simulink subsystem "AirframePowertrain"  (R2024b)
settings: Solver=VariableStepAuto  StartTime=0.0  StopTime=10.0  RelTol=1e-3
undefined symbols (not defined in the file): contact, motorPID, percWeightGain, uavParam, windVel
libraries: mbdriLib x3, aerolibasang x2, fl_lib x1, nesl_utility x1
settings Model: Creator=jjha  LastModifiedBy=jjha
settings RTWCC: GPUComputeCapability=3.5

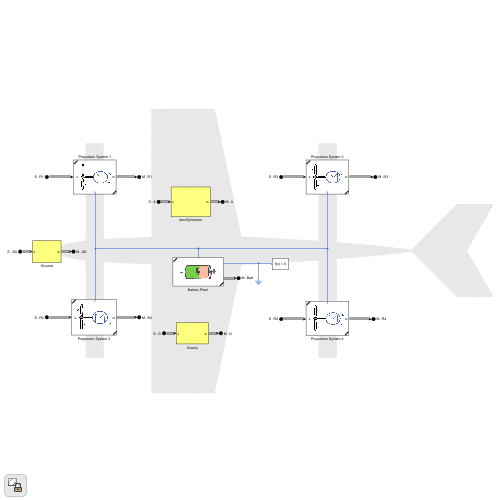
[thumbnail: Simulink's stored preview of the top-level diagram]
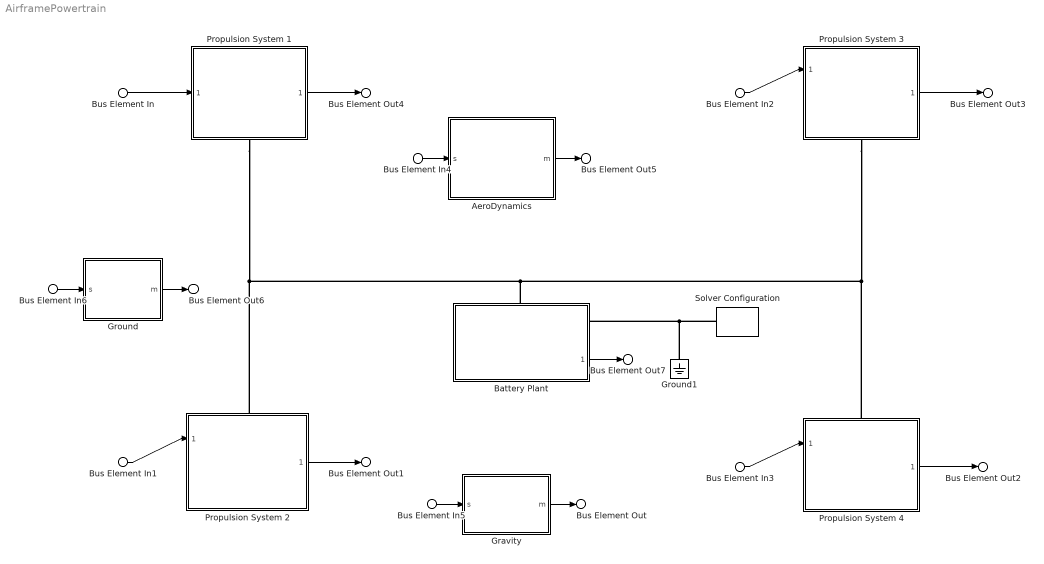
== system AirframePowertrain ==
  Bus Element In : Inport  PortName=S  Element=R1
  Bus Element In1 : Inport  PortName=S  Element=R2
  Bus Element In2 : Inport  PortName=S  Element=R3
  Bus Element In3 : Inport  PortName=S  Element=R4
  Bus Element In4 : Inport  PortName=S  Element=A
  Bus Element In5 : Inport  PortName=S  Element=G
  Bus Element In6 : Inport  PortName=S  Element=AD
  AeroDynamics : Subsystem
  Battery Plant : Subsystem  ReferencedSubsystem=BatteryPlantModel_Table
      settings: PortSchema="{\"entries\":[{\"content\":{\"sides\":[{\"content\":{\"connectorIds\":[\"LConn1\"]},\"type\":\"ConnectorPlacement.EquallySpacedRectSide\",\"uuid\":\"ba36f307-b33b-4535-ba0b-2e0bfd99fc4d\"},{\"content\":{\"connectorIds\":[\"RConn2\",\"Out1\"],\"side\":\"RIGHT\"},\"type\":\"ConnectorPlacement.EquallySpacedRectSide\",\"uuid\":\"89704593-04c2-4c1a-a3b9-13b3f56a74b5\"},{\"content\":{\"connectorIds\":[\"RConn1\"],\"side\":\"TOP\"},\"type\":\"ConnectorPlacement.EquallySpacedRectSide\",\"uuid\":\"1daeac74-7d2b-4aa4-8837-06dc1649b516\"},{\"content\":{\"side\":\"BOTTOM\"},\"type\":\"ConnectorPlacement.EquallySpacedRectSide\",\"uuid\":\"a55355a8-f534-49c8-a897-d3f7ff506222\"}]},\"type\":\"ConnectorPlacement.EquallySpacedConnector\",\"uuid\":\"2c693ef8-3b08-48d7-935c-b55223a280fc\"}],\"packageUris\":[\"http://schema.mathworks.com/mf0/Connector/R2020b\"],\"version\":\"1.0\"}"
  Gravity : Subsystem
  Ground : Subsystem
  Ground1 : fl_lib/Electrical/Electrical Elements/Electrical Reference
  Propulsion System 1 : Subsystem  ReferencedSubsystem=PropulsionSystem  RotorArm=uavParam.geom.RotorArm1  Kp=motorPID.Kpp  Ki=motorPID.Kii  Kd=motorPID.Kdd  N=motorPID.N
      settings: PortSchema="{\"entries\":[{\"content\":{\"sides\":[{\"content\":{\"connectorIds\":[\"In1\"]},\"type\":\"ConnectorPlacement.EquallySpacedRectSide\",\"uuid\":\"a75aafe4-98d2-4ab0-9654-1a116df6472c\"},{\"content\":{\"connectorIds\":[\"Out1\"],\"side\":\"RIGHT\"},\"type\":\"ConnectorPlacement.EquallySpacedRectSide\",\"uuid\":\"2075eb3f-d81d-4e0c-b871-39ed3a8467db\"},{\"content\":{\"side\":\"TOP\"},\"type\":\"ConnectorPlacement.EquallySpacedRectSide\",\"uuid\":\"9db392e5-d372-4f9a-b849-10c0fd16bebf\"},{\"content\":{\"connectorIds\":[\"RConn1\"],\"side\":\"BOTTOM\"},\"type\":\"ConnectorPlacement.EquallySpacedRectSide\",\"uuid\":\"0cb625c0-fbe4-4004-9810-4dcf6ffdfbe8\"}]},\"type\":\"ConnectorPlacement.EquallySpacedConnector\",\"uuid\":\"a89763ad-9d11-48f7-8f0c-3b7b7595f410\"}],\"packageUris\":[\"http://schema.mathworks.com/mf0/Connector/R2020b\"],\"version\":\"1.0\"}"
  Propulsion System 2 : Subsystem  ReferencedSubsystem=PropulsionSystem  RotorArm=uavParam.geom.RotorArm2  Kp=motorPID.Kpp  Ki=motorPID.Kii  Kd=motorPID.Kdd  N=motorPID.N
      settings: PortSchema="{\"entries\":[{\"content\":{\"sides\":[{\"content\":{\"connectorIds\":[\"In1\",\"LConn1\"]},\"type\":\"ConnectorPlacement.EquallySpacedRectSide\",\"uuid\":\"a75aafe4-98d2-4ab0-9654-1a116df6472c\"},{\"content\":{\"connectorIds\":[\"Out1\"],\"side\":\"RIGHT\"},\"type\":\"ConnectorPlacement.EquallySpacedRectSide\",\"uuid\":\"2075eb3f-d81d-4e0c-b871-39ed3a8467db\"},{\"content\":{\"connectorIds\":[\"RConn1\"],\"side\":\"TOP\"},\"type\":\"ConnectorPlacement.EquallySpacedRectSide\",\"uuid\":\"9db392e5-d372-4f9a-b849-10c0fd16bebf\"}]},\"type\":\"ConnectorPlacement.EquallySpacedConnector\",\"uuid\":\"a89763ad-9d11-48f7-8f0c-3b7b7595f410\"}],\"packageUris\":[\"http://schema.mathworks.com/mf0/Connector/R2020b\"],\"version\":\"1.0\"}"
  Propulsion System 3 : Subsystem  ReferencedSubsystem=PropulsionSystem  RotorArm=uavParam.geom.RotorArm3  Kp=motorPID.Kpp  Ki=motorPID.Kii  Kd=motorPID.Kdd  N=motorPID.N
      settings: PortSchema="{\"entries\":[{\"content\":{\"sides\":[{\"content\":{\"connectorIds\":[\"In1\",\"LConn1\"]},\"type\":\"ConnectorPlacement.EquallySpacedRectSide\",\"uuid\":\"a75aafe4-98d2-4ab0-9654-1a116df6472c\"},{\"content\":{\"connectorIds\":[\"Out1\"],\"side\":\"RIGHT\"},\"type\":\"ConnectorPlacement.EquallySpacedRectSide\",\"uuid\":\"2075eb3f-d81d-4e0c-b871-39ed3a8467db\"},{\"content\":{\"side\":\"TOP\"},\"type\":\"ConnectorPlacement.EquallySpacedRectSide\",\"uuid\":\"9db392e5-d372-4f9a-b849-10c0fd16bebf\"},{\"content\":{\"connectorIds\":[\"RConn1\"],\"side\":\"BOTTOM\"},\"type\":\"ConnectorPlacement.EquallySpacedRectSide\",\"uuid\":\"14e310fc-3705-44ea-ab02-95783124972c\"}]},\"type\":\"ConnectorPlacement.EquallySpacedConnector\",\"uuid\":\"a89763ad-9d11-48f7-8f0c-3b7b7595f410\"}],\"packageUris\":[\"http://schema.mathworks.com/mf0/Connector/R2020b\"],\"version\":\"1.0\"}"
  Propulsion System 4 : Subsystem  ReferencedSubsystem=PropulsionSystem  RotorArm=uavParam.geom.RotorArm4  Kp=motorPID.Kpp  Ki=motorPID.Kii  Kd=motorPID.Kdd  N=motorPID.N
      settings: PortSchema="{\"entries\":[{\"content\":{\"sides\":[{\"content\":{\"connectorIds\":[\"In1\",\"LConn1\"]},\"type\":\"ConnectorPlacement.EquallySpacedRectSide\",\"uuid\":\"a75aafe4-98d2-4ab0-9654-1a116df6472c\"},{\"content\":{\"connectorIds\":[\"Out1\"],\"side\":\"RIGHT\"},\"type\":\"ConnectorPlacement.EquallySpacedRectSide\",\"uuid\":\"2075eb3f-d81d-4e0c-b871-39ed3a8467db\"},{\"content\":{\"connectorIds\":[\"RConn1\"],\"side\":\"TOP\"},\"type\":\"ConnectorPlacement.EquallySpacedRectSide\",\"uuid\":\"9db392e5-d372-4f9a-b849-10c0fd16bebf\"}]},\"type\":\"ConnectorPlacement.EquallySpacedConnector\",\"uuid\":\"a89763ad-9d11-48f7-8f0c-3b7b7595f410\"}],\"packageUris\":[\"http://schema.mathworks.com/mf0/Connector/R2020b\"],\"version\":\"1.0\"}"
  Solver Configuration : nesl_utility/Solver Configuration  PhysicalDomain=network_engine_domain  SubClassName=solver  LeftPortType=input  RightPortType=generic  Tones=[]  Harmonics=[]  SimulateNoise=off  Profile=off  UseLocalSampling=off  EnableSwitchedLinearOptims=on  FrequencyDomain=off  UseCCode=off  RelTol=0.001  AbsTol=0.001  MinStep=1e-09  ToWorkspace=off  RevertToSquareIcSolve=off  NumHomotopyIterations=100  PhasorMode=off  PhasorModeNumHarmonics=1  ConsistencySolver=NEWTON_XTOL_AFTER_FTOL  IndexReductionMethod=DerivativeReplacement  DoDC=off  ResidualTolerance=1e-09  ConsistencyTolSource=GLOBAL  ConsistencyAbsTol=0.001  ConsistencyRelTol=0.001  ConsistencyTolFactor=0.001  UseLocalSolver=on  LocalSolverChoice=NE_BACKWARD_EULER_ADVANCER  ResolveIndetEquations=on  FunctionEvalNumThread=1  LocalSolverSampleTime=0.01  DoFixedCost=off  MaxNonlinIter=3  MaxModeIter=2  ComputeImpulses=off  ImpulseIterations=2  LinearAlgebra=auto  LinearAlgebraNumThread=0  EquationFormulation=NE_TIME_EF  DelaysMemoryBudget=1024  AutomaticFiltering=on  FilteringTimeConstant=0.001  PartitionStorageMethod=AS_NEEDED  PartitionMemoryBudget=1024  PartitionMethod=ROBUST  MultibodyUseLocalSolver=off  MultibodyLocalSolverChoice=ODE1  MultibodyLocalSolverSampleTime=0.001
  Bus Element Out : Outport  PortName=M  Element=G
  Bus Element Out1 : Outport  PortName=M  Element=R2
  Bus Element Out2 : Outport  PortName=M  Element=R4
  Bus Element Out3 : Outport  PortName=M  Element=R3
  Bus Element Out4 : Outport  PortName=M  Element=R1
  Bus Element Out5 : Outport  PortName=M  Element=A
  Bus Element Out6 : Outport  PortName=M  Element=AD
  Bus Element Out7 : Outport  PortName=M  Element=Batt
  wires:
  Bus Element In1/1 -> Propulsion System 2/1
  Bus Element In2/1 -> Propulsion System 3/1
  Bus Element In3/1 -> Propulsion System 4/1
  Bus Element In/1 -> Propulsion System 1/1
  Bus Element In4/1 -> AeroDynamics/1(s)
  Bus Element In5/1 -> Gravity/1(s)
  Gravity/1(m) -> Bus Element Out/1
  Propulsion System 2/1 -> Bus Element Out1/1
  Propulsion System 4/1 -> Bus Element Out2/1
  Propulsion System 3/1 -> Bus Element Out3/1
  Propulsion System 1/1 -> Bus Element Out4/1
  AeroDynamics/1(m) -> Bus Element Out5/1
  Bus Element In6/1 -> Ground/1(s)
  Ground/1(m) -> Bus Element Out6/1
  Battery Plant/1 -> Bus Element Out7/1
  connections:
  Propulsion System 3/RConn1 -- Propulsion System 1/RConn1 -- Propulsion System 2/RConn1 -- Battery Plant/RConn1 -- Propulsion System 4/RConn1
  Solver Configuration/RConn1 -- Ground1/LConn1 -- Battery Plant/RConn2

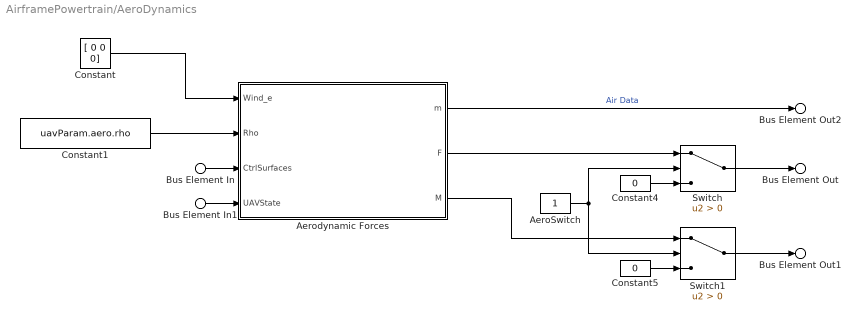
== system AirframePowertrain/AeroDynamics ==
  Bus Element In : Inport  PortName=s  Element=Ctrl
  Bus Element In1 : Inport  PortName=s  Element=St
  AeroSwitch : Constant
  Aerodynamic Forces : Subsystem
  Constant : Constant  Value=[ 0 0 0]
      settings: AttributesFormatString=%<Value>
  Constant1 : Constant  Value=uavParam.aero.rho
  Constant4 : Constant  Value=0
  Constant5 : Constant  Value=0
  Switch : Switch  Criteria=u2 > Threshold  SaturateOnIntegerOverflow=off  InputSameDT=off
  Switch1 : Switch  Criteria=u2 > Threshold  SaturateOnIntegerOverflow=off  InputSameDT=off
  Bus Element Out : Outport  PortName=m  Element=Force
  Bus Element Out1 : Outport  PortName=m  Element=Moment
  Bus Element Out2 : Outport  PortName=m  Element=AirData
  wires:
  Bus Element In1/1 -> Aerodynamic Forces/4(UAVState)
  Bus Element In/1 -> Aerodynamic Forces/3(CtrlSurfaces)
  Constant4/1 -> Switch/3
  Aerodynamic Forces/3(M) -> Switch1/1
  Aerodynamic Forces/2(F) -> Switch/1
  Constant5/1 -> Switch1/3
  AeroSwitch/1 -> Switch/2, Switch1/2
  Constant/1 -> Aerodynamic Forces/1(Wind_e)
  Constant1/1 -> Aerodynamic Forces/2(Rho)
  Aerodynamic Forces/1(m) -> Bus Element Out2/1  "Air Data"
  Switch/1 -> Bus Element Out/1
  Switch1/1 -> Bus Element Out1/1

== system AirframePowertrain/Gravity ==
  Bus Element In : Inport  PortName=s  Element=DCMbe
  Constant : Constant  Value=[0 0 uavParam.aero.g]'
  Gain : Gain  Gain=uavParam.geom.mass*percWeightGain
  Matrix Multiply : Product  Multiplication=Matrix(*)
  Bus Element Out : Outport  PortName=m  Element=gravityForce
  wires:
  Bus Element In/1 -> Matrix Multiply/1
  Constant/1 -> Matrix Multiply/2
  Matrix Multiply/1 -> Gain/1
  Gain/1 -> Bus Element Out/1  "Gravity Force"

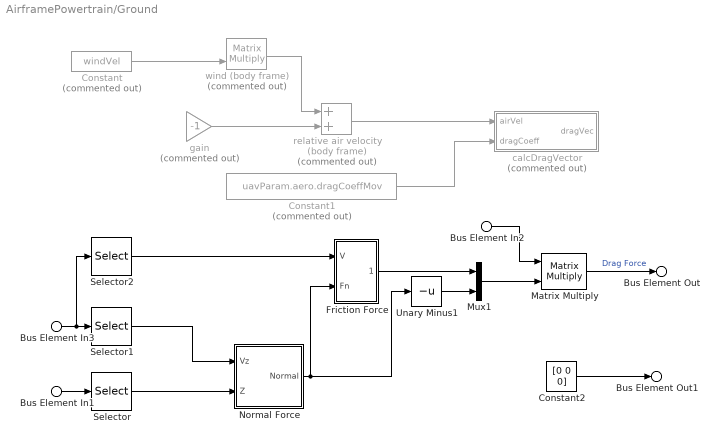
== system AirframePowertrain/Ground ==
  Bus Element In2 : Inport  PortName=s  Element=DCMbe
  Bus Element In3 : Inport  PortName=s  Element=Ve
  Bus Element In1 : Inport  PortName=s  Element=Xe
  Constant : Constant  Commented=on  Value=windVel
  Constant1 : Constant  Commented=on  Value=uavParam.aero.dragCoeffMov
  Constant2 : Constant  Value=[0 0 0]  SampleTime=-1
  Friction Force : Subsystem
  Matrix Multiply : Product  Multiplication=Matrix(*)
  Mux1 : Mux  Inputs=2
  Normal Force : Subsystem
  Selector : Selector  InputPortWidth=3  IndexOptions=Index vector (dialog)  Indices=[3]  OutputSizes=1
  Selector1 : Selector  InputPortWidth=3  IndexOptions=Index vector (dialog)  Indices=[3]  OutputSizes=1
  Selector2 : Selector  InputPortWidth=3  IndexOptions=Index vector (dialog)  Indices=[1,2]  OutputSizes=1
  Unary Minus1 : UnaryMinus
  calcDragVector : MATLAB Function  Commented=on  TreatAsAtomicUnit=on
  gain : Gain  Commented=on  Gain=-1
  relative air velocity (body frame) : Sum  Commented=on
  wind (body frame) : Product  Commented=on  Multiplication=Matrix(*)
  Bus Element Out : Outport  PortName=m  Element=GroundForce
  Bus Element Out1 : Outport  PortName=m  Element=GroundMoment
  wires:
  Normal Force/1(Normal) -> Unary Minus1/1, Friction Force/2(Fn)
  Selector1/1 -> Normal Force/1(Vz)
  Constant2/1 -> Bus Element Out1/1
  Selector/1 -> Normal Force/2(Z)
  Unary Minus1/1 -> Mux1/2
  Bus Element In1/1 -> Selector/1
  Mux1/1 -> Matrix Multiply/2
  Friction Force/1(Friction) -> Mux1/1
  Bus Element In2/1 -> Matrix Multiply/1
  Bus Element In3/1 -> Selector1/1, Selector2/1
  Selector2/1 -> Friction Force/1(V)
  ? -> gain/1
  relative air velocity (body frame)/1 -> calcDragVector/1(airVel)
  gain/1 -> relative air velocity (body frame)/2
  Constant1/1 -> calcDragVector/2(dragCoeff)
  Constant/1 -> wind (body frame)/2
  wind (body frame)/1 -> relative air velocity (body frame)/1
  Matrix Multiply/1 -> Bus Element Out/1  "Drag Force"

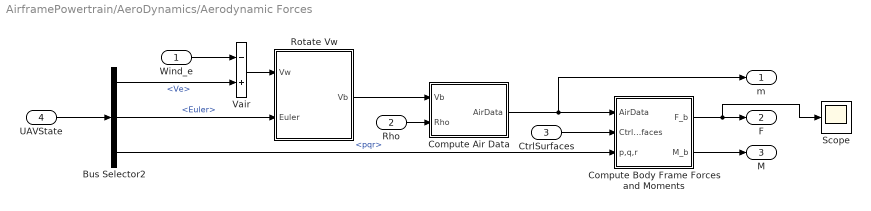
== system AirframePowertrain/AeroDynamics/Aerodynamic Forces ==
  Wind_e : Inport
  Rho : Inport  Port=2
  CtrlSurfaces : Inport  Port=3
  UAVState : Inport  Port=4
  Bus Selector2 : BusSelector  OutputSignals=Ve,Euler,pqr
  Compute Air Data : Subsystem  TreatAsAtomicUnit=on  VariantControl=use_aerospace_blocks == 1
  Compute Body Frame Forces and Moments : Subsystem
  Rotate Vw : Subsystem
  Scope : Scope
  Vair : Sum  Inputs=-+  InputSameDT=on  SaturateOnIntegerOverflow=on  OutDataTypeStr=Inherit: Same as first input
  m : Outport  VectorParamsAs1DForOutWhenUnconnected=off
  F : Outport  Port=2
  M : Outport  Port=3
  wires:
  Vair/1 -> Rotate Vw/1(Vw)
  Bus Selector2/2 -> Rotate Vw/2(Euler)  "<Euler>"
  Rho/1 -> Compute Air Data/2(Rho)
  Rotate Vw/1(Vb) -> Compute Air Data/1(Vb)
  Compute Body Frame Forces and Moments/2(M_b) -> M/1
  Bus Selector2/3 -> Compute Body Frame Forces and Moments/3(p,q,r)  "<pqr>"
  Compute Air Data/1(AirData) -> Compute Body Frame Forces and Moments/1(AirData), m/1
  CtrlSurfaces/1 -> Compute Body Frame Forces and Moments/2(CtrlSurfaces)
  Wind_e/1 -> Vair/1
  Compute Body Frame Forces and Moments/1(F_b) -> F/1, Scope/1
  UAVState/1 -> Bus Selector2/1
  Bus Selector2/1 -> Vair/2  "<Ve>"

== system AirframePowertrain/Ground/Friction Force ==
  V : Inport
  Fn : Inport  Port=2
  Product : Product
  Soft Coulomb Friction : Subsystem
  Unary Minus : UnaryMinus
  Friction : Outport
  wires:
  V/1 -> Soft Coulomb Friction/1(V)
  Product/1 -> Unary Minus/1
  Soft Coulomb Friction/1(Out1) -> Product/1
  Fn/1 -> Product/2
  Unary Minus/1 -> Friction/1

== system AirframePowertrain/Ground/Normal Force ==
  Vz : Inport
  Z : Inport  Port=2
  Add : Sum
  Constant : Constant  Value=0  SampleTime=-1
  Damper : Gain  Gain=-sqrt(contact.spring*uavParam.geom.mass)
  Saturation : Saturate  UpperLimit=inf  LowerLimit=0  ZeroCross=off
  Spring Kp : Gain  Gain=-contact.spring
  Switch : Switch  Criteria=u2 > Threshold  SaturateOnIntegerOverflow=off  InputSameDT=off
  Unary Minus : UnaryMinus
  Unary Minus1 : UnaryMinus
  Normal : Outport
  wires:
  Unary Minus1/1 -> Damper/1
  Unary Minus/1 -> Switch/2, Spring Kp/1
  Saturation/1 -> Normal/1
  Vz/1 -> Unary Minus1/1
  Spring Kp/1 -> Add/1
  Damper/1 -> Add/2
  Switch/1 -> Saturation/1
  Z/1 -> Unary Minus/1
  Constant/1 -> Switch/1
  Add/1 -> Switch/3

== system AirframePowertrain/AeroDynamics/Aerodynamic Forces/Compute Air Data ==
  Vb : Inport  PortDimensions=3
  Rho : Inport  Port=2
  Add : Sum
  Bus Creator : BusCreator  Inputs=4
  Constant : Constant  Value=5/57.296
  Dynamic Pressure : aerolibasang/Dynamic Pressure
  Gain : Gain
  "Incidence, Sideslip, & Airspeed" : aerolibasang/Incidence, Sideslip, & Airspeed
  Saturation : Saturate  UpperLimit=14*pi/180  LowerLimit=-14*pi/180
  To Workspace : ToWorkspace  VariableName=Alpha  SaveFormat=Timeseries  SampleTime=-1
  AirData : Outport  VectorParamsAs1DForOutWhenUnconnected=off
  wires:
  Add/1 -> Gain/1  "alpha"
  Gain/1 -> To Workspace/1
  Constant/1 -> Add/1
  "Incidence, Sideslip, & Airspeed"/1 -> Bus Creator/1, Add/2  "alpha"
  Saturation/1 -> Bus Creator/2  "beta"
  "Incidence, Sideslip, & Airspeed"/2 -> Saturation/1  "beta"
  Vb/1 -> Dynamic Pressure/1, "Incidence, Sideslip, & Airspeed"/1
  Dynamic Pressure/1 -> Bus Creator/4  "q"
  "Incidence, Sideslip, & Airspeed"/3 -> Bus Creator/3  "airspeed"
  Rho/1 -> Dynamic Pressure/2
  Bus Creator/1 -> AirData/1

== system AirframePowertrain/AeroDynamics/Aerodynamic Forces/Compute Body Frame Forces and Moments ==
  AirData : Inport
  CtrlSurfaces : Inport  Port=2
  p,q,r : Inport  Port=3
  Bus Selector : BusSelector  OutputSignals=alpha,beta
  Mux : Mux  Inputs=2
  Rotate FM to body frame : Subsystem
  Wind frame F& M : Subsystem
  F_b : Outport  Unit=kg*m/s^2  VectorParamsAs1DForOutWhenUnconnected=off
  M_b : Outport  Port=2  Unit=kg*m/s  VectorParamsAs1DForOutWhenUnconnected=off
  wires:
  AirData/1 -> Bus Selector/1, Wind frame F& M/1(Airdata)
  CtrlSurfaces/1 -> Wind frame F& M/2(CtrlSurfaces)
  Rotate FM to body frame/1(F_b) -> F_b/1
  Rotate FM to body frame/2(M_b) -> M_b/1
  p,q,r/1 -> Wind frame F& M/3(p,q,r)
  Wind frame F& M/1(FM_w) -> Rotate FM to body frame/1(FM_w)  "FM_W"
  Bus Selector/1 -> Mux/1  "<alpha>"
  Bus Selector/2 -> Mux/2  "<beta>"
  Mux/1 -> Rotate FM to body frame/2(alpha_beta)

== system AirframePowertrain/AeroDynamics/Aerodynamic Forces/Rotate Vw ==
  Vw : Inport
  Euler : Inport  Port=2
  RL2B : mbdriLib/Coordinates/RL2B  SystemSampleTime=-1  VariantActivationTime=update diagram  AllowFlexibleInterface=on  Latency=0  AutoFrameSizeCalculation=off
  RL2B * Vw : Product  Multiplication=Matrix(*)  InputSameDT=on  SaturateOnIntegerOverflow=on  OutDataTypeStr=Inherit: Same as first input
  Vb : Outport  Unit=m/s  VectorParamsAs1DForOutWhenUnconnected=off
  wires:
  Euler/1 -> RL2B/1
  RL2B/1 -> RL2B * Vw/1
  Vw/1 -> RL2B * Vw/2
  RL2B * Vw/1 -> Vb/1

== system AirframePowertrain/Ground/Friction Force/Soft Coulomb Friction ==
  note: Pennestrì, E., Rossi, V., Salvini, P. et al. Review and comparison of dry friction force models. Nonlinear Dyn 83, 1785–1801 (2016). https://doi.org/10.1007/s11071-015-2485-3
  V : Inport
  Tanh : Trigonometry  Operator=tanh
  friction coefficient : Gain  Gain=contact.rollingFriction*1.2
  vd : Gain  Gain=1/contact.vd
  Out1 : Outport
  wires:
  friction coefficient/1 -> Out1/1
  Tanh/1 -> friction coefficient/1
  vd/1 -> Tanh/1
  V/1 -> vd/1

== system AirframePowertrain/AeroDynamics/Aerodynamic Forces/Compute Body Frame Forces and Moments/Rotate FM to body frame ==
  FM_w : Inport
  alpha_beta : Inport  Port=2
  Forces : Selector  InputPortWidth=6  IndexOptions=Index vector (dialog)  Indices=[1 2 3]  OutputSizes=[(-2)]
  Moments : Selector  InputPortWidth=6  IndexOptions=Index vector (dialog)  Indices=[4 5 6]  OutputSizes=[(-2)]
  Rotate Forces : Subsystem
  Rotate Moments : Subsystem
  F_b : Outport  VectorParamsAs1DForOutWhenUnconnected=off
  M_b : Outport  Port=2  VectorParamsAs1DForOutWhenUnconnected=off
  wires:
  Rotate Forces/1(F_b) -> F_b/1
  Rotate Moments/1(M_b) -> M_b/1
  Forces/1 -> Rotate Forces/1(F_w)
  FM_w/1 -> Forces/1, Moments/1
  Moments/1 -> Rotate Moments/2(M_w)
  alpha_beta/1 -> Rotate Moments/1(alpha_beta), Rotate Forces/2(alpha_beta)

== system AirframePowertrain/AeroDynamics/Aerodynamic Forces/Compute Body Frame Forces and Moments/Wind frame F& M ==
  Airdata : Inport
  CtrlSurfaces : Inport  Port=2
  p,q,r : Inport  Port=3
  Bus Creator1 : BusCreator  Inputs=2
  Bus Selector1 : BusSelector  OutputSignals=dA,dR
  Bus Selector2 : BusSelector  OutputSignals=dE,dA,dR
  Bus Selector6 : BusSelector  OutputSignals=beta,airspeed
  Bus Selector7 : BusSelector  OutputSignals=alpha,airspeed
  Get Forces and Moments : Subsystem
  Lateral Channel : Subsystem
  Longitudinal Channel : Subsystem
  FM_w : Outport  PortDimensions=6  VectorParamsAs1DForOutWhenUnconnected=off
  wires:
  Bus Selector2/3 -> Longitudinal Channel/6(dR)  "<dR>"
  Bus Selector2/2 -> Longitudinal Channel/5(dA)  "<dA>"
  Longitudinal Channel/1(Longitudinal) -> Bus Creator1/2
  Lateral Channel/1(Lateral) -> Bus Creator1/1
  p,q,r/1 -> Longitudinal Channel/4(p,q,r), Lateral Channel/5(p,q,r)
  CtrlSurfaces/1 -> Bus Selector2/1, Bus Selector1/1
  Bus Selector1/1 -> Lateral Channel/3(dA)  "<dA>"
  Bus Selector1/2 -> Lateral Channel/4(dR)  "<dR>"
  Bus Selector2/1 -> Longitudinal Channel/3(dE)  "<dE>"
  Airdata/1 -> Get Forces and Moments/1(Airdata), Bus Selector7/1, Bus Selector6/1
  Bus Selector6/1 -> Lateral Channel/1(beta)  "<beta>"
  Bus Selector6/2 -> Lateral Channel/2(Airspeed)  "<airspeed>"
  Bus Selector7/1 -> Longitudinal Channel/1(alpha)  "<alpha>"
  Bus Selector7/2 -> Longitudinal Channel/2(Airpseed)  "<airspeed>"
  Bus Creator1/1 -> Get Forces and Moments/2(AeroCoeffs)
  Get Forces and Moments/1(FM_w) -> FM_w/1

== system AirframePowertrain/AeroDynamics/Aerodynamic Forces/Compute Body Frame Forces and Moments/Rotate FM to body frame/Rotate Forces ==
  F_w : Inport
  alpha_beta : Inport  Port=2
  Product2 : Product  Multiplication=Matrix(*)  SaturateOnIntegerOverflow=on  OutDataTypeStr=Inherit: Same as first input
  RB2W : Subsystem
  RW2B : Math  Operator=transpose  SignedPower=on
  F_b : Outport  PortDimensions=3  VectorParamsAs1DForOutWhenUnconnected=off
  wires:
  RB2W/1(Rw2b) -> RW2B/1
  alpha_beta/1 -> RB2W/1(aoa beta)
  Product2/1 -> F_b/1
  F_w/1 -> Product2/2
  RW2B/1 -> Product2/1

== system AirframePowertrain/AeroDynamics/Aerodynamic Forces/Compute Body Frame Forces and Moments/Rotate FM to body frame/Rotate Moments ==
  alpha_beta : Inport
  M_w : Inport  Port=2
  Product2 : Product  Multiplication=Matrix(*)  SaturateOnIntegerOverflow=on  OutDataTypeStr=Inherit: Same as first input
  RB2W : Subsystem
  RW2B : Math  Operator=transpose  SignedPower=on
  M_b : Outport  PortDimensions=3  VectorParamsAs1DForOutWhenUnconnected=off
  wires:
  M_w/1 -> Product2/2
  Product2/1 -> M_b/1
  alpha_beta/1 -> RB2W/1(aoa beta)
  RB2W/1(Rw2b) -> RW2B/1
  RW2B/1 -> Product2/1

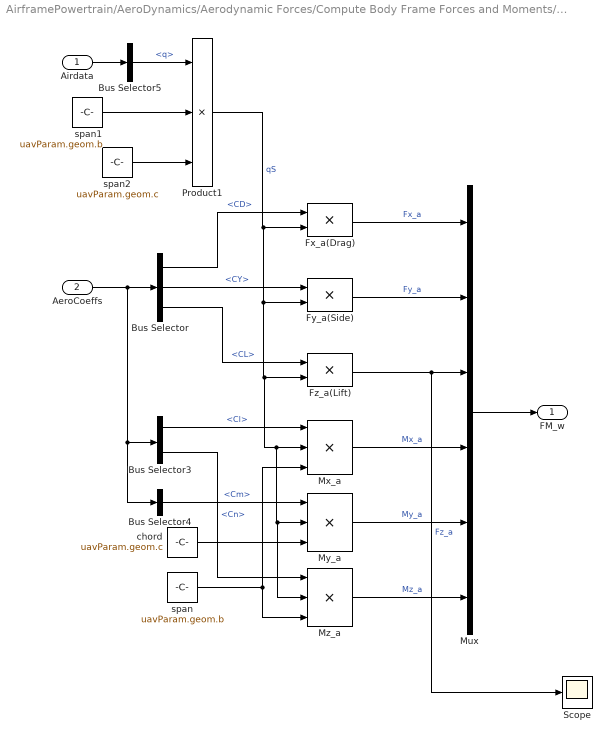
== system AirframePowertrain/AeroDynamics/Aerodynamic Forces/Compute Body Frame Forces and Moments/Wind frame F& M/Get Forces and Moments ==
  Airdata : Inport
  AeroCoeffs : Inport  Port=2
  Bus Selector : BusSelector  OutputSignals=signal2.CD,signal1.CY,signal2.CL
  Bus Selector3 : BusSelector  OutputSignals=signal1.Cl,signal1.Cn
  Bus Selector4 : BusSelector  OutputSignals=signal2.Cm
  Bus Selector5 : BusSelector  OutputSignals=q
  Fx_a(Drag) : Product  Inputs=**  SaturateOnIntegerOverflow=on  OutDataTypeStr=Inherit: Same as first input
  Fy_a(Side) : Product  SaturateOnIntegerOverflow=on  OutDataTypeStr=Inherit: Same as first input
  Fz_a(Lift) : Product  SaturateOnIntegerOverflow=on  OutDataTypeStr=Inherit: Same as first input
  Mux : Mux  Inputs=6
  Mx_a : Product  Inputs=3  SaturateOnIntegerOverflow=on  OutDataTypeStr=Inherit: Same as first input
  My_a : Product  Inputs=3  SaturateOnIntegerOverflow=on  OutDataTypeStr=Inherit: Same as first input
  Mz_a : Product  Inputs=3  SaturateOnIntegerOverflow=on  OutDataTypeStr=Inherit: Same as first input
  Product1 : Product  Inputs=3  SaturateOnIntegerOverflow=on  OutDataTypeStr=Inherit: Same as first input
  Scope : Scope
  chord : Constant  Value=uavParam.geom.c  VectorParams1D=off
      settings: AttributesFormatString=%<Value>
  span : Constant  Value=uavParam.geom.b  VectorParams1D=off
      settings: AttributesFormatString=%<Value>
  span1 : Constant  Value=uavParam.geom.b  VectorParams1D=off
      settings: AttributesFormatString=%<Value>
  span2 : Constant  Value=uavParam.geom.c  VectorParams1D=off
      settings: AttributesFormatString=%<Value>
  FM_w : Outport  VectorParamsAs1DForOutWhenUnconnected=off
  wires:
  Bus Selector5/1 -> Product1/1  "<q>"
  Bus Selector3/1 -> Mx_a/1  "<Cl>"
  span1/1 -> Product1/2
  Product1/1 -> Mz_a/2, My_a/2, Mx_a/2, Fz_a(Lift)/2, Fy_a(Side)/2, Fx_a(Drag)/2  "qS"
  Bus Selector/3 -> Fz_a(Lift)/1  "<CL>"
  Bus Selector3/2 -> Mz_a/1  "<Cn>"
  Mux/1 -> FM_w/1
  Fy_a(Side)/1 -> Mux/2  "Fy_a"
  span/1 -> Mx_a/3, Mz_a/3
  chord/1 -> My_a/3
  Airdata/1 -> Bus Selector5/1
  Mz_a/1 -> Mux/6  "Mz_a"
  Fz_a(Lift)/1 -> Mux/3, Scope/1  "Fz_a"
  My_a/1 -> Mux/5  "My_a"
  AeroCoeffs/1 -> Bus Selector3/1, Bus Selector4/1, Bus Selector/1
  Bus Selector/1 -> Fx_a(Drag)/1  "<CD>"
  Fx_a(Drag)/1 -> Mux/1  "Fx_a"
  span2/1 -> Product1/3
  Bus Selector4/1 -> My_a/1  "<Cm>"
  Bus Selector/2 -> Fy_a(Side)/1  "<CY>"
  Mx_a/1 -> Mux/4  "Mx_a"

== system AirframePowertrain/AeroDynamics/Aerodynamic Forces/Compute Body Frame Forces and Moments/Wind frame F& M/Lateral Channel ==
  beta : Inport
  Airspeed : Inport  Port=2
  dA : Inport  Port=3
  dR : Inport  Port=4
  p,q,r : Inport  Port=5
  Bus Creator : BusCreator  Inputs=3
  CY : Subsystem
  Cl : Subsystem
  Cn : Subsystem
  Lateral : Outport  VectorParamsAs1DForOutWhenUnconnected=off
  wires:
  Bus Creator/1 -> Lateral/1
  CY/1(CY) -> Bus Creator/1  "CY"
  Cn/1(Cn) -> Bus Creator/3  "Cn"
  beta/1 -> Cn/1(beta), Cl/1(beta), CY/1(beta)
  dA/1 -> Cn/2(dA), Cl/2(dA)
  dR/1 -> Cn/3(dR), Cl/3(dR), CY/2(dR)
  Airspeed/1 -> Cl/5(Airspeed), Cn/5(Airspeed), CY/4(Airspeed)
  p,q,r/1 -> CY/3(p,q,r), Cl/4(p,q,r), Cn/4(p,q,r)
  Cl/1(Cl) -> Bus Creator/2  "Cl"

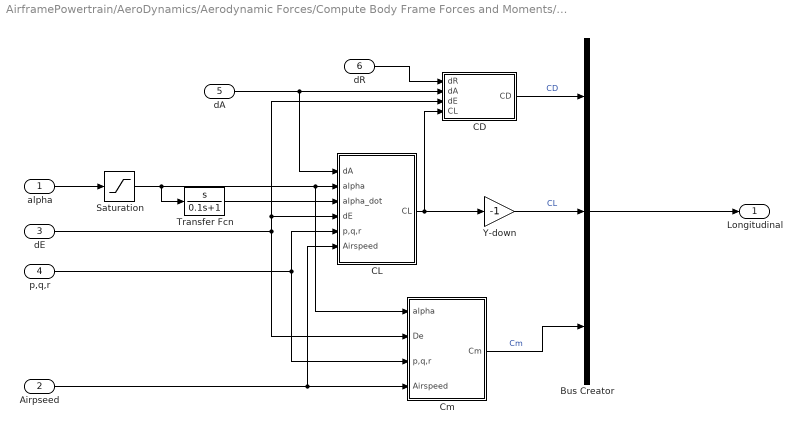
== system AirframePowertrain/AeroDynamics/Aerodynamic Forces/Compute Body Frame Forces and Moments/Wind frame F& M/Longitudinal Channel ==
  alpha : Inport
  Airpseed : Inport  Port=2
  dE : Inport  Port=3
  p,q,r : Inport  Port=4
  dA : Inport  Port=5
  dR : Inport  Port=6
  Bus Creator : BusCreator  Inputs=3
  CD : Subsystem
  CL : Subsystem
  Cm : Subsystem
  Saturation : Saturate  UpperLimit=14*pi/180  LowerLimit=-14*pi/180
  Transfer Fcn : TransferFcn  Numerator=[1 0]  Denominator=[0.1 1]
  Y-down : Gain  Gain=-1  SaturateOnIntegerOverflow=on  OutDataTypeStr=Inherit: Same as input  ParamDataTypeStr=Inherit: Same as input
      settings: AttributesFormatString=%<Gain>
  Longitudinal : Outport  VectorParamsAs1DForOutWhenUnconnected=off
  wires:
  Saturation/1 -> Cm/1(alpha), CL/2(alpha), Transfer Fcn/1
  dA/1 -> CD/2(dA), CL/1(dA)
  dR/1 -> CD/1(dR)
  alpha/1 -> Saturation/1
  CD/1(CD) -> Bus Creator/1  "CD"
  Y-down/1 -> Bus Creator/2  "CL"
  dE/1 -> Cm/2(De), CL/4(dE), CD/3(dE)
  CL/1(CL) -> CD/4(CL), Y-down/1
  Cm/1(Cm) -> Bus Creator/3  "Cm"
  Bus Creator/1 -> Longitudinal/1
  p,q,r/1 -> Cm/3(p,q,r), CL/5(p,q,r)
  Airpseed/1 -> Cm/4(Airspeed), CL/6(Airspeed)
  Transfer Fcn/1 -> CL/3(alpha_dot)

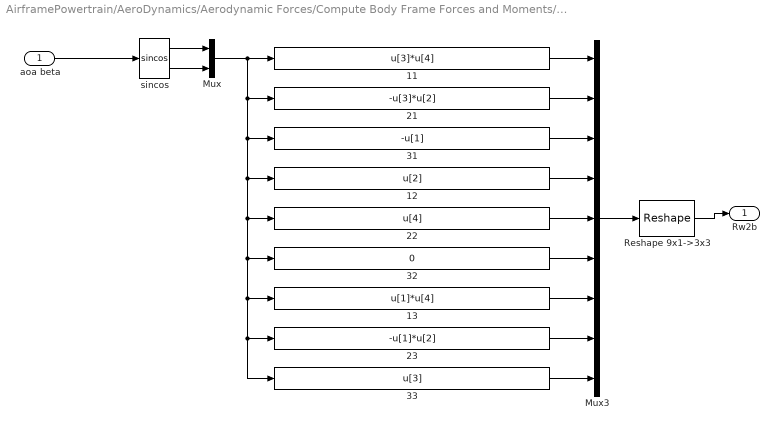
== system AirframePowertrain/AeroDynamics/Aerodynamic Forces/Compute Body Frame Forces and Moments/Rotate FM to body frame/Rotate Forces/RB2W ==
  aoa beta : Inport
  11 : Fcn  Expr=u[3]*u[4]
  12 : Fcn  Expr=u[2]
  13 : Fcn  Expr=u[1]*u[4]
  21 : Fcn  Expr=-u[3]*u[2]
  22 : Fcn  Expr=u[4]
  23 : Fcn  Expr=-u[1]*u[2]
  31 : Fcn  Expr=-u[1]
  32 : Fcn  Expr=0
  33 : Fcn  Expr=u[3]
  Mux : Mux  Inputs=2
  Mux3 : Mux  Inputs=9
  Reshape 9x1->3x3 : Reshape  OutputDimensionality=Customize  OutputDimensions=[3,3]
  sincos : Trigonometry  Operator=sincos
  Rw2b : Outport  VectorParamsAs1DForOutWhenUnconnected=off
  wires:
  Mux3/1 -> Reshape 9x1->3x3/1
  Reshape 9x1->3x3/1 -> Rw2b/1
  11/1 -> Mux3/1
  21/1 -> Mux3/2
  31/1 -> Mux3/3
  12/1 -> Mux3/4
  22/1 -> Mux3/5
  32/1 -> Mux3/6
  13/1 -> Mux3/7
  23/1 -> Mux3/8
  33/1 -> Mux3/9
  sincos/1 -> Mux/1
  sincos/2 -> Mux/2
  aoa beta/1 -> sincos/1
  Mux/1 -> 33/1, 23/1, 13/1, 32/1, 22/1, 12/1, 31/1, 21/1, 11/1

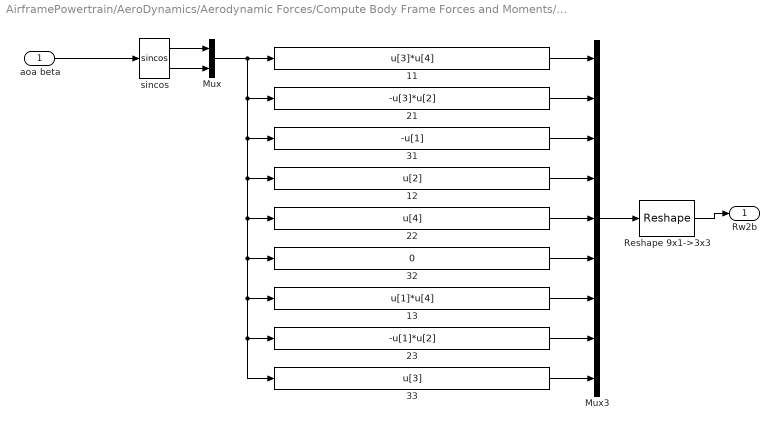
== system AirframePowertrain/AeroDynamics/Aerodynamic Forces/Compute Body Frame Forces and Moments/Rotate FM to body frame/Rotate Moments/RB2W ==
  aoa beta : Inport
  11 : Fcn  Expr=u[3]*u[4]
  12 : Fcn  Expr=u[2]
  13 : Fcn  Expr=u[1]*u[4]
  21 : Fcn  Expr=-u[3]*u[2]
  22 : Fcn  Expr=u[4]
  23 : Fcn  Expr=-u[1]*u[2]
  31 : Fcn  Expr=-u[1]
  32 : Fcn  Expr=0
  33 : Fcn  Expr=u[3]
  Mux : Mux  Inputs=2
  Mux3 : Mux  Inputs=9
  Reshape 9x1->3x3 : Reshape  OutputDimensionality=Customize  OutputDimensions=[3,3]
  sincos : Trigonometry  Operator=sincos
  Rw2b : Outport  VectorParamsAs1DForOutWhenUnconnected=off
  wires:
  Mux3/1 -> Reshape 9x1->3x3/1
  Reshape 9x1->3x3/1 -> Rw2b/1
  11/1 -> Mux3/1
  21/1 -> Mux3/2
  31/1 -> Mux3/3
  12/1 -> Mux3/4
  22/1 -> Mux3/5
  32/1 -> Mux3/6
  13/1 -> Mux3/7
  23/1 -> Mux3/8
  33/1 -> Mux3/9
  sincos/1 -> Mux/1
  sincos/2 -> Mux/2
  aoa beta/1 -> sincos/1
  Mux/1 -> 33/1, 23/1, 13/1, 32/1, 22/1, 12/1, 31/1, 21/1, 11/1

== system AirframePowertrain/AeroDynamics/Aerodynamic Forces/Compute Body Frame Forces and Moments/Wind frame F& M/Lateral Channel/CY ==
  beta : Inport
  dR : Inport  Port=2
  p,q,r : Inport  Port=3
  Airspeed : Inport  Port=4
  CYDr : Constant  Value=uavParam.aero.CYDr
      settings: AttributesFormatString=%<Value>
  CYb : Constant  Value=uavParam.aero.CYb
      settings: AttributesFormatString=%<Value>
  Product : Product  SaturateOnIntegerOverflow=on  OutDataTypeStr=Inherit: Same as first input
  Product1 : Product  SaturateOnIntegerOverflow=on  OutDataTypeStr=Inherit: Same as first input
  Sum2 : Sum  Inputs=++++  SaturateOnIntegerOverflow=on
  roll factors : Subsystem
  CY : Outport  VectorParamsAs1DForOutWhenUnconnected=off
  wires:
  roll factors/2(CYr) -> Sum2/4
  roll factors/1(CYp) -> Sum2/3
  p,q,r/1 -> roll factors/1(p,q,r)
  Airspeed/1 -> roll factors/2(Airspeed)
  Sum2/1 -> CY/1
  CYb/1 -> Product/1
  beta/1 -> Product/2
  Product/1 -> Sum2/1
  CYDr/1 -> Product1/1
  dR/1 -> Product1/2
  Product1/1 -> Sum2/2

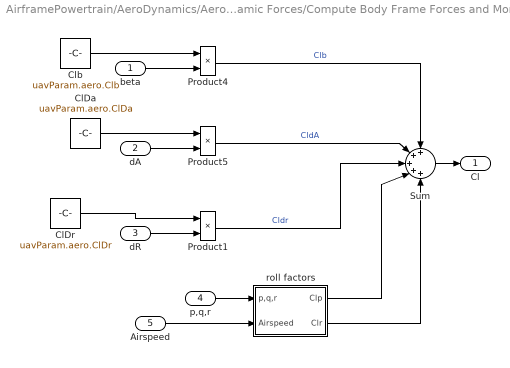
== system AirframePowertrain/AeroDynamics/Aerodynamic Forces/Compute Body Frame Forces and Moments/Wind frame F& M/Lateral Channel/Cl ==
  beta : Inport
  dA : Inport  Port=2
  dR : Inport  Port=3
  p,q,r : Inport  Port=4
  Airspeed : Inport  Port=5
  ClDa : Constant  Value=uavParam.aero.ClDa
      settings: AttributesFormatString=%<Value>
  ClDr : Constant  Value=uavParam.aero.ClDr
      settings: AttributesFormatString=%<Value>
  Clb : Constant  Value=uavParam.aero.Clb
      settings: AttributesFormatString=%<Value>
  Product1 : Product  SaturateOnIntegerOverflow=on  OutDataTypeStr=Inherit: Same as first input
  Product4 : Product  SaturateOnIntegerOverflow=on  OutDataTypeStr=Inherit: Same as first input
  Product5 : Product  SaturateOnIntegerOverflow=on  OutDataTypeStr=Inherit: Same as first input
  Sum : Sum  Inputs=+++++  SaturateOnIntegerOverflow=on
  roll factors : Subsystem
  Cl : Outport  VectorParamsAs1DForOutWhenUnconnected=off
  wires:
  Clb/1 -> Product4/1
  beta/1 -> Product4/2
  ClDa/1 -> Product5/1
  dA/1 -> Product5/2
  ClDr/1 -> Product1/1
  dR/1 -> Product1/2
  Sum/1 -> Cl/1
  Product4/1 -> Sum/1  "Clb"
  Product1/1 -> Sum/3  "Cldr"
  roll factors/2(Clr) -> Sum/5
  p,q,r/1 -> roll factors/1(p,q,r)
  Airspeed/1 -> roll factors/2(Airspeed)
  Product5/1 -> Sum/2  "CldA"
  roll factors/1(Clp) -> Sum/4

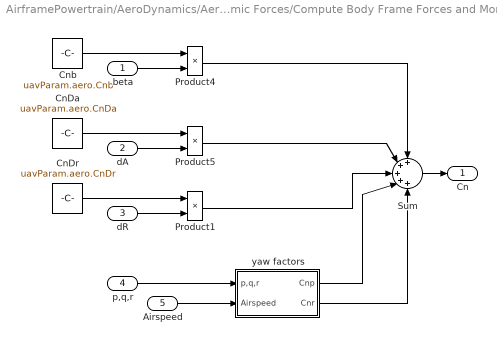
== system AirframePowertrain/AeroDynamics/Aerodynamic Forces/Compute Body Frame Forces and Moments/Wind frame F& M/Lateral Channel/Cn ==
  beta : Inport
  dA : Inport  Port=2
  dR : Inport  Port=3
  p,q,r : Inport  Port=4
  Airspeed : Inport  Port=5
  CnDa : Constant  Value=uavParam.aero.CnDa
      settings: AttributesFormatString=%<Value>
  CnDr : Constant  Value=uavParam.aero.CnDr
      settings: AttributesFormatString=%<Value>
  Cnb : Constant  Value=uavParam.aero.Cnb
      settings: AttributesFormatString=%<Value>
  Product1 : Product  SaturateOnIntegerOverflow=on  OutDataTypeStr=Inherit: Same as first input
  Product4 : Product  SaturateOnIntegerOverflow=on  OutDataTypeStr=Inherit: Same as first input
  Product5 : Product  SaturateOnIntegerOverflow=on  OutDataTypeStr=Inherit: Same as first input
  Sum : Sum  Inputs=+++++  SaturateOnIntegerOverflow=on
  yaw factors : Subsystem
  Cn : Outport  VectorParamsAs1DForOutWhenUnconnected=off
  wires:
  Product4/1 -> Sum/1
  yaw factors/1(Cnp) -> Sum/4
  yaw factors/2(Cnr) -> Sum/5
  Product1/1 -> Sum/3
  Sum/1 -> Cn/1
  dR/1 -> Product1/2
  CnDr/1 -> Product1/1
  dA/1 -> Product5/2
  Product5/1 -> Sum/2
  CnDa/1 -> Product5/1
  beta/1 -> Product4/2
  Cnb/1 -> Product4/1
  p,q,r/1 -> yaw factors/1(p,q,r)
  Airspeed/1 -> yaw factors/2(Airspeed)

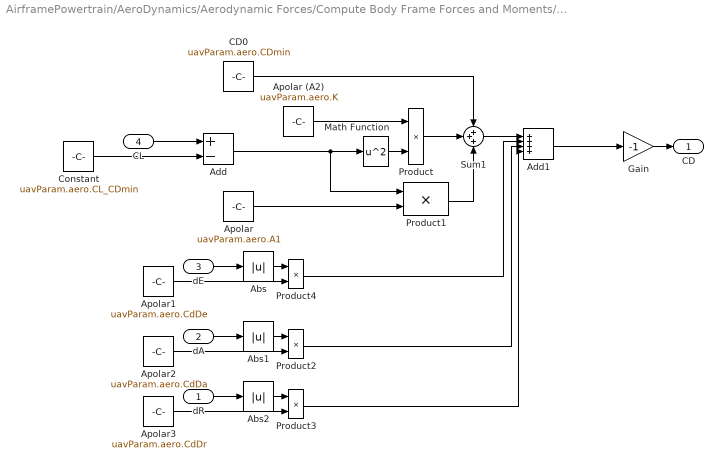
== system AirframePowertrain/AeroDynamics/Aerodynamic Forces/Compute Body Frame Forces and Moments/Wind frame F& M/Longitudinal Channel/CD ==
  dR : Inport
  dA : Inport  Port=2
  dE : Inport  Port=3
  CL : Inport  Port=4
  Abs : Abs  SaturateOnIntegerOverflow=off
  Abs1 : Abs  SaturateOnIntegerOverflow=off
  Abs2 : Abs  SaturateOnIntegerOverflow=off
  Add : Sum  Inputs=+-
  Add1 : Sum  Inputs=++++
  Apolar : Constant  Value=uavParam.aero.A1
      settings: AttributesFormatString=%<Value>
  Apolar (A2) : Constant  Value=uavParam.aero.K
      settings: AttributesFormatString=%<Value>
  Apolar1 : Constant  Value=uavParam.aero.CdDe
      settings: AttributesFormatString=%<Value>
  Apolar2 : Constant  Value=uavParam.aero.CdDa
      settings: AttributesFormatString=%<Value>
  Apolar3 : Constant  Value=uavParam.aero.CdDr
      settings: AttributesFormatString=%<Value>
  CD0 : Constant  Value=uavParam.aero.CDmin
      settings: AttributesFormatString=%<Value>
  Constant : Constant  Value=uavParam.aero.CL_CDmin
  Gain : Gain  Gain=-1  SaturateOnIntegerOverflow=on  OutDataTypeStr=Inherit: Same as input  ParamDataTypeStr=Inherit: Same as input
      settings: AttributesFormatString=%<Gain>
  Math Function : Math  Operator=square  SignedPower=on
  Product{,1..4} (5 alike) : Product  SaturateOnIntegerOverflow=on  OutDataTypeStr=Inherit: Same as first input
  Sum1 : Sum  Inputs=+++  SaturateOnIntegerOverflow=on
  CD : Outport  VectorParamsAs1DForOutWhenUnconnected=off
  wires:
  Product3/1 -> Add1/4
  Product2/1 -> Add1/3
  Product4/1 -> Add1/2
  Add1/1 -> Gain/1
  Sum1/1 -> Add1/1
  dR/1 -> Abs2/1
  Apolar3/1 -> Product3/2
  Abs2/1 -> Product3/1
  dA/1 -> Abs1/1
  Apolar2/1 -> Product2/2
  Abs1/1 -> Product2/1
  Abs/1 -> Product4/1
  dE/1 -> Abs/1
  Apolar1/1 -> Product4/2
  Constant/1 -> Add/2
  CL/1 -> Add/1
  Apolar/1 -> Product1/2
  CD0/1 -> Sum1/1
  Add/1 -> Math Function/1, Product1/1
  Product/1 -> Sum1/2
  Product1/1 -> Sum1/3
  Math Function/1 -> Product/2
  Apolar (A2)/1 -> Product/1
  Gain/1 -> CD/1

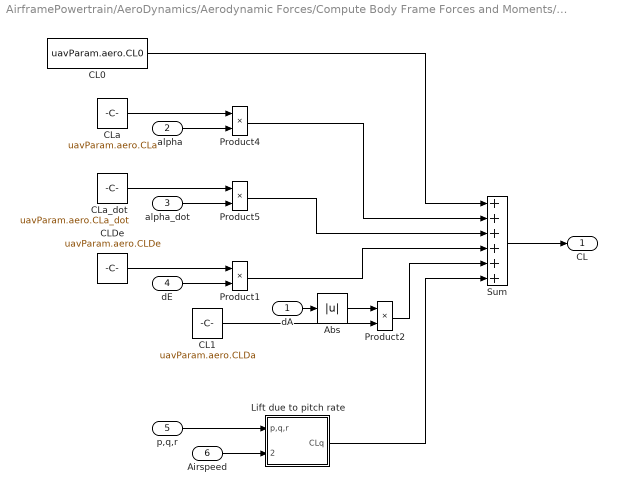
== system AirframePowertrain/AeroDynamics/Aerodynamic Forces/Compute Body Frame Forces and Moments/Wind frame F& M/Longitudinal Channel/CL ==
  dA : Inport
  alpha : Inport  Port=2
  alpha_dot : Inport  Port=3
  dE : Inport  Port=4
  p,q,r : Inport  Port=5
  Airspeed : Inport  Port=6
  Abs : Abs  SaturateOnIntegerOverflow=off
  CL0 : Constant  Value=uavParam.aero.CL0
      settings: AttributesFormatString=%<Value>
  CL1 : Constant  Value=uavParam.aero.CLDa
      settings: AttributesFormatString=%<Value>
  CLDe : Constant  Value=uavParam.aero.CLDe
      settings: AttributesFormatString=%<Value>
  CLa : Constant  Value=uavParam.aero.CLa
      settings: AttributesFormatString=%<Value>
  CLa_dot : Constant  Value=uavParam.aero.CLa_dot
      settings: AttributesFormatString=%<Value>
  Lift due to pitch rate : Subsystem
  Product{1..2,4..5} (4 alike) : Product  SaturateOnIntegerOverflow=on  OutDataTypeStr=Inherit: Same as first input
  Sum : Sum  Inputs=++++++  SaturateOnIntegerOverflow=on
  CL : Outport  VectorParamsAs1DForOutWhenUnconnected=off
  wires:
  Abs/1 -> Product2/1
  dA/1 -> Abs/1
  Product2/1 -> Sum/5
  CL1/1 -> Product2/2
  Lift due to pitch rate/1(CLq) -> Sum/6
  Product4/1 -> Sum/2
  CLa/1 -> Product4/1
  alpha/1 -> Product4/2
  CLa_dot/1 -> Product5/1
  alpha_dot/1 -> Product5/2
  CLDe/1 -> Product1/1
  dE/1 -> Product1/2
  Sum/1 -> CL/1
  Product5/1 -> Sum/3
  Product1/1 -> Sum/4
  p,q,r/1 -> Lift due to pitch rate/1(p,q,r)
  Airspeed/1 -> Lift due to pitch rate/2(Airspeed)
  CL0/1 -> Sum/1

== system AirframePowertrain/AeroDynamics/Aerodynamic Forces/Compute Body Frame Forces and Moments/Wind frame F& M/Longitudinal Channel/Cm ==
  alpha : Inport
  De : Inport  Port=2
  p,q,r : Inport  Port=3
  Airspeed : Inport  Port=4
  Cm0 : Constant  Value=uavParam.aero.Cm0
      settings: AttributesFormatString=%<Value>
  CmDe : Constant  Value=uavParam.aero.CmDe
      settings: AttributesFormatString=%<Value>
  Cma : Constant  Value=uavParam.aero.Cma
      settings: AttributesFormatString=%<Value>
  Lift due to pitch rate : Subsystem
  Product1 : Product  Inputs=**  SaturateOnIntegerOverflow=on  OutDataTypeStr=Inherit: Same as first input
  Product4 : Product  SaturateOnIntegerOverflow=on  OutDataTypeStr=Inherit: Same as first input
  Sum : Sum  Inputs=++++  SaturateOnIntegerOverflow=on
  Cm : Outport  VectorParamsAs1DForOutWhenUnconnected=off
  wires:
  alpha/1 -> Product4/2
  Airspeed/1 -> Lift due to pitch rate/2(Airspeed)
  Cm0/1 -> Sum/1  "cm0"
  Cma/1 -> Product4/1
  CmDe/1 -> Product1/1
  De/1 -> Product1/2
  Sum/1 -> Cm/1  "total"
  Product4/1 -> Sum/2  "cma"
  Product1/1 -> Sum/3  "cmde"
  p,q,r/1 -> Lift due to pitch rate/1(p,q,r)
  Lift due to pitch rate/1(Cmq) -> Sum/4  "cmq"

== system AirframePowertrain/AeroDynamics/Aerodynamic Forces/Compute Body Frame Forces and Moments/Wind frame F& M/Lateral Channel/CY/roll factors ==
  p,q,r : Inport
  Airspeed : Inport  Port=2
  Constant : Constant  Value=uavParam.aero.CYp
      settings: AttributesFormatString=%<Value>
  Constant1 : Constant  Value=uavParam.aero.CYr
      settings: AttributesFormatString=%<Value>
  Get p : Selector  InputPortWidth=3  IndexOptions=Index vector (dialog)  Indices=1  OutputSizes=[(-2)]
  Get r : Selector  InputPortWidth=3  IndexOptions=Index vector (dialog)  Indices=3  OutputSizes=[(-2)]
  Product : Product  SaturateOnIntegerOverflow=on  OutDataTypeStr=Inherit: Same as first input
  Product1 : Product  SaturateOnIntegerOverflow=on  OutDataTypeStr=Inherit: Same as first input
  Subsystem : Subsystem
  roll rate fact : Subsystem
  CYp : Outport  VectorParamsAs1DForOutWhenUnconnected=off
  CYr : Outport  Port=2  VectorParamsAs1DForOutWhenUnconnected=off
  wires:
  Product/1 -> CYp/1
  Product1/1 -> CYr/1
  Constant/1 -> Product/1
  roll rate fact/1(Roll Rate Fac) -> Product/2
  Constant1/1 -> Product1/1
  Subsystem/1(Yaw Rate Fac) -> Product1/2
  Airspeed/1 -> roll rate fact/2(Airspeed), Subsystem/2(Airspeed)
  Get p/1 -> roll rate fact/1(p)
  p,q,r/1 -> Get p/1, Get r/1
  Get r/1 -> Subsystem/1(r)

== system AirframePowertrain/AeroDynamics/Aerodynamic Forces/Compute Body Frame Forces and Moments/Wind frame F& M/Lateral Channel/Cl/roll factors ==
  p,q,r : Inport
  Airspeed : Inport  Port=2
  Constant : Constant  Value=uavParam.aero.Clp
      settings: AttributesFormatString=%<Value>
  Constant1 : Constant  Value=uavParam.aero.Clr
      settings: AttributesFormatString=%<Value>
  Get p : Selector  InputPortWidth=3  IndexOptions=Index vector (dialog)  Indices=1  OutputSizes=[(-2)]
  Get r : Selector  InputPortWidth=3  IndexOptions=Index vector (dialog)  Indices=3  OutputSizes=[(-2)]
  Product : Product  SaturateOnIntegerOverflow=on  OutDataTypeStr=Inherit: Same as first input
  Product1 : Product  SaturateOnIntegerOverflow=on  OutDataTypeStr=Inherit: Same as first input
  roll rate fact : Subsystem
  yaw rate fact : mbdriLib/Utilities/yaw rate fact  SystemSampleTime=-1  VariantActivationTime=update diagram  AllowFlexibleInterface=on  Latency=0  AutoFrameSizeCalculation=off
  Clp : Outport  VectorParamsAs1DForOutWhenUnconnected=off
  Clr : Outport  Port=2  VectorParamsAs1DForOutWhenUnconnected=off
  wires:
  Product/1 -> Clp/1
  Product1/1 -> Clr/1
  Constant/1 -> Product/1
  roll rate fact/1(Roll Rate Fac) -> Product/2
  Constant1/1 -> Product1/1
  yaw rate fact/1 -> Product1/2
  Airspeed/1 -> roll rate fact/2(Airspeed), yaw rate fact/2
  Get p/1 -> roll rate fact/1(p)
  p,q,r/1 -> Get p/1, Get r/1
  Get r/1 -> yaw rate fact/1

== system AirframePowertrain/AeroDynamics/Aerodynamic Forces/Compute Body Frame Forces and Moments/Wind frame F& M/Lateral Channel/Cn/yaw factors ==
  p,q,r : Inport
  Airspeed : Inport  Port=2
  Constant : Constant  Value=uavParam.aero.Cnp
      settings: AttributesFormatString=%<Value>
  Constant1 : Constant  Value=uavParam.aero.Cnr
      settings: AttributesFormatString=%<Value>
  Get p : Selector  InputPortWidth=3  IndexOptions=Index vector (dialog)  Indices=1  OutputSizes=[(-2)]
  Get r : Selector  InputPortWidth=3  IndexOptions=Index vector (dialog)  Indices=3  OutputSizes=[(-2)]
  Product : Product  SaturateOnIntegerOverflow=on  OutDataTypeStr=Inherit: Same as first input
  Product1 : Product  SaturateOnIntegerOverflow=on  OutDataTypeStr=Inherit: Same as first input
  roll rate fact : Subsystem
  yaw rate fact : mbdriLib/Utilities/yaw rate fact  SystemSampleTime=-1  VariantActivationTime=update diagram  AllowFlexibleInterface=on  Latency=0  AutoFrameSizeCalculation=off
  Cnp : Outport  VectorParamsAs1DForOutWhenUnconnected=off
  Cnr : Outport  Port=2  VectorParamsAs1DForOutWhenUnconnected=off
  wires:
  Product/1 -> Cnp/1
  Product1/1 -> Cnr/1
  Constant1/1 -> Product1/1
  yaw rate fact/1 -> Product1/2
  Constant/1 -> Product/1
  roll rate fact/1(Roll Rate Fac) -> Product/2
  Get p/1 -> roll rate fact/1(p)
  p,q,r/1 -> Get p/1, Get r/1
  Get r/1 -> yaw rate fact/1
  Airspeed/1 -> roll rate fact/2(Airspeed), yaw rate fact/2

== system AirframePowertrain/AeroDynamics/Aerodynamic Forces/Compute Body Frame Forces and Moments/Wind frame F& M/Longitudinal Channel/CL/Lift due to pitch rate ==
  p,q,r : Inport
  Airspeed : Inport  Port=2
  Constant : Constant  Value=uavParam.aero.CLq
      settings: AttributesFormatString=%<Value>
  Get q : Selector  InputPortWidth=3  IndexOptions=Index vector (dialog)  Indices=2  OutputSizes=[(-2)]
  Product : Product  SaturateOnIntegerOverflow=on  OutDataTypeStr=Inherit: Same as first input
  pitch rate factor : Subsystem
  CLq : Outport  VectorParamsAs1DForOutWhenUnconnected=off
  wires:
  Constant/1 -> Product/1
  pitch rate factor/1(Pitch Rate Fac) -> Product/2
  Product/1 -> CLq/1
  p,q,r/1 -> Get q/1
  Get q/1 -> pitch rate factor/1(q)
  Airspeed/1 -> pitch rate factor/2(Airspeed)

== system AirframePowertrain/AeroDynamics/Aerodynamic Forces/Compute Body Frame Forces and Moments/Wind frame F& M/Longitudinal Channel/Cm/Lift due to pitch rate ==
  p,q,r : Inport
  Airspeed : Inport  Port=2
  Constant : Constant  Value=uavParam.aero.Cmq
      settings: AttributesFormatString=%<Value>
  Get q : Selector  InputPortWidth=3  IndexOptions=Index vector (dialog)  Indices=2  OutputSizes=[(-2)]
  Product : Product  SaturateOnIntegerOverflow=on  OutDataTypeStr=Inherit: Same as first input
  pitch rate factor : Subsystem
  Cmq : Outport  VectorParamsAs1DForOutWhenUnconnected=off
  wires:
  Constant/1 -> Product/1
  pitch rate factor/1(Pitch Rate Fac) -> Product/2
  Product/1 -> Cmq/1
  p,q,r/1 -> Get q/1
  Get q/1 -> pitch rate factor/1(q)
  Airspeed/1 -> pitch rate factor/2(Airspeed)

== system AirframePowertrain/AeroDynamics/Aerodynamic Forces/Compute Body Frame Forces and Moments/Wind frame F& M/Lateral Channel/CY/roll factors/Subsystem ==
  r : Inport
  Airspeed : Inport  Port=2
  Cmq3 : Constant
      settings: AttributesFormatString=%<Value>
  Cmq4 : Constant  Value=uavParam.geom.b
      settings: AttributesFormatString=%<Value>
  Gain : Gain  Gain=2
  Product1 : Product  Inputs=***/  SaturateOnIntegerOverflow=on  OutDataTypeStr=Inherit: Same as first input
  Saturation : Saturate  UpperLimit=inf  LowerLimit=0.1
      settings: AttributesFormatString="[%<LowerLimit>  %<UpperLimit>]"
  Yaw Rate Fac : Outport  VectorParamsAs1DForOutWhenUnconnected=off
  wires:
  r/1 -> Product1/1
  Product1/1 -> Yaw Rate Fac/1
  Cmq3/1 -> Product1/2
  Gain/1 -> Product1/4
  Airspeed/1 -> Saturation/1
  Cmq4/1 -> Product1/3
  Saturation/1 -> Gain/1

== system AirframePowertrain/AeroDynamics/Aerodynamic Forces/Compute Body Frame Forces and Moments/Wind frame F& M/Lateral Channel/CY/roll factors/roll rate fact ==
  p : Inport
  Airspeed : Inport  Port=2
  Cmq1 : Constant
      settings: AttributesFormatString=%<Value>
  Cmq2 : Constant  Value=uavParam.geom.b
      settings: AttributesFormatString=%<Value>
  Gain : Gain  Gain=2
  Product : Product  Inputs=***/  SaturateOnIntegerOverflow=on  OutDataTypeStr=Inherit: Same as first input
  Saturation : Saturate  UpperLimit=inf  LowerLimit=0.1
      settings: AttributesFormatString="[%<LowerLimit>  %<UpperLimit>]"
  Roll Rate Fac : Outport  VectorParamsAs1DForOutWhenUnconnected=off
  wires:
  Gain/1 -> Product/4
  Saturation/1 -> Gain/1
  Product/1 -> Roll Rate Fac/1
  p/1 -> Product/1
  Cmq1/1 -> Product/2
  Cmq2/1 -> Product/3
  Airspeed/1 -> Saturation/1

== system AirframePowertrain/AeroDynamics/Aerodynamic Forces/Compute Body Frame Forces and Moments/Wind frame F& M/Lateral Channel/Cl/roll factors/roll rate fact ==
  p : Inport
  Airspeed : Inport  Port=2
  Cmq1 : Constant  Value=.5
      settings: AttributesFormatString=%<Value>
  Cmq2 : Constant  Value=uavParam.geom.b
      settings: AttributesFormatString=%<Value>
  Product : Product  Inputs=***/  SaturateOnIntegerOverflow=on  OutDataTypeStr=Inherit: Same as first input
  Saturation : Saturate  UpperLimit=inf  LowerLimit=0.1
      settings: AttributesFormatString="[%<LowerLimit>  %<UpperLimit>]"
  Roll Rate Fac : Outport  VectorParamsAs1DForOutWhenUnconnected=off
  wires:
  Product/1 -> Roll Rate Fac/1
  p/1 -> Product/1
  Cmq1/1 -> Product/2
  Cmq2/1 -> Product/3
  Airspeed/1 -> Saturation/1
  Saturation/1 -> Product/4

== system AirframePowertrain/AeroDynamics/Aerodynamic Forces/Compute Body Frame Forces and Moments/Wind frame F& M/Lateral Channel/Cn/yaw factors/roll rate fact ==
  p : Inport
  Airspeed : Inport  Port=2
  Cmq1 : Constant  Value=.5
      settings: AttributesFormatString=%<Value>
  Cmq2 : Constant  Value=uavParam.geom.b
      settings: AttributesFormatString=%<Value>
  Product : Product  Inputs=***/  SaturateOnIntegerOverflow=on  OutDataTypeStr=Inherit: Same as first input
  Saturation : Saturate  UpperLimit=inf  LowerLimit=0.1
      settings: AttributesFormatString="[%<LowerLimit>  %<UpperLimit>]"
  Roll Rate Fac : Outport  VectorParamsAs1DForOutWhenUnconnected=off
  wires:
  Product/1 -> Roll Rate Fac/1
  p/1 -> Product/1
  Cmq1/1 -> Product/2
  Cmq2/1 -> Product/3
  Airspeed/1 -> Saturation/1
  Saturation/1 -> Product/4

== system AirframePowertrain/AeroDynamics/Aerodynamic Forces/Compute Body Frame Forces and Moments/Wind frame F& M/Longitudinal Channel/CL/Lift due to pitch rate/pitch rate factor ==
  q : Inport
  Airspeed : Inport  Port=2
  Cmq2 : Constant  Value=uavParam.geom.c
      settings: AttributesFormatString=%<Value>
  Gain : Gain  Gain=2
  Product : Product  Inputs=**/  SaturateOnIntegerOverflow=on  OutDataTypeStr=Inherit: Same as first input
  Saturation : Saturate  UpperLimit=inf  LowerLimit=0.1
      settings: AttributesFormatString="[%<LowerLimit>  %<UpperLimit>]"
  Pitch Rate Fac : Outport  VectorParamsAs1DForOutWhenUnconnected=off
  wires:
  Gain/1 -> Product/3
  Saturation/1 -> Gain/1
  Product/1 -> Pitch Rate Fac/1
  q/1 -> Product/1
  Airspeed/1 -> Saturation/1
  Cmq2/1 -> Product/2

== system AirframePowertrain/AeroDynamics/Aerodynamic Forces/Compute Body Frame Forces and Moments/Wind frame F& M/Longitudinal Channel/Cm/Lift due to pitch rate/pitch rate factor ==
  q : Inport
  Airspeed : Inport  Port=2
  Cmq2 : Constant  Value=uavParam.geom.c
      settings: AttributesFormatString=%<Value>
  Gain : Gain  Gain=2
  Product : Product  Inputs=**/  SaturateOnIntegerOverflow=on  OutDataTypeStr=Inherit: Same as first input
  Saturation : Saturate  UpperLimit=inf  LowerLimit=0.1
      settings: AttributesFormatString="[%<LowerLimit>  %<UpperLimit>]"
  Pitch Rate Fac : Outport  VectorParamsAs1DForOutWhenUnconnected=off
  wires:
  Gain/1 -> Product/3
  Saturation/1 -> Gain/1
  Product/1 -> Pitch Rate Fac/1
  q/1 -> Product/1
  Airspeed/1 -> Saturation/1
  Cmq2/1 -> Product/2

== matlab function AirframePowertrain/Ground/calcDragVector ==
  data: airVel input; dragVec output; dragCoeff input
function dragVec = fcn(airVel, dragCoeff)

dragVec = dragCoeff * norm(airVel) * airVel;

end
